simulink model "tenzoRobustV1"  (Simulink 7.9)
settings: Solver=ode23s  StartTime=0.0  StopTime=15  RelTol=1e-3
values from neighbouring files (symbols this model uses):
  AMI = AK1    [AstaTenzoV3.m]
  AMin = [ ... (first row only)    [AstaTenzoV3.m]
  Aoss = AMin-V*ClocalMin    [AstaTenzoV3.m]
  BMI = BK1    [AstaTenzoV3.m]
  ClocalMin = [ ... (first row only)    [AstaTenzoV3.m]
  CMI = eye(q*mu)    [AstaTenzoV3.m]
  Coss = eye(n)    [AstaTenzoV3.m]
  D_phi = [1 325.437715018286 23852.1596168943 0]    [AstaTenzoV3.m]
  D_psi = [1 378.139322580724 35127.9961825618 0]    [AstaTenzoV3.m]
  D_theta = [1 325.437715018286 23852.1596168943 0]    [AstaTenzoV3.m]
  D_thrust = [1 963.786798861645 190423.384445206 0]    [AstaTenzoV3.m]
  DMI = zeros(q*mu,q)    [AstaTenzoV3.m]
  Dmod = [N D]    [AstaTenzoV3.m]
  Doss = zeros(size(Bossw))    [AstaTenzoV3.m]
  F1 = F(:,size(AMin,1)+1:size(F,2))    [AstaTenzoV3.m]
  F2 = F(:,1:size(AMin,1))    [AstaTenzoV3.m]
  k1 = 1    [AstaTenzoV3.m]
  k2 = 1.869    [AstaTenzoV3.m]
  k3 = 2.002    [AstaTenzoV3.m]
  k4 = 1.996    [AstaTenzoV3.m]
  Kt = ct*rho*rp^4*pi()    [AstaTenzoV3.m]
  Ktm = Km/Kt    [AstaTenzoV3.m]
  lx = 28.8e-3    (= 0.0288)    [AstaTenzoV3.m]
  ly = 28.8e-3    (= 0.0288)    [AstaTenzoV3.m]
  N_phi = [440.513056398418 26779.6272064186          272303.182447317 584729.91630594]    [AstaTenzoV3.m]
  N_psi = [59260.0621820611 3429565.45270113           27702908.9364068 53625940.9126871]    [AstaTenzoV3.m]
  N_theta = [440.513056398418 26779.6272064186          272303.182447317 584729.91630594]    [AstaTenzoV3.m]
  N_thrust = [682900.887332905 4668183.15145263]    [AstaTenzoV3.m]
  omega = 0.5    [AstaTenzoV3.m]
  tc = 0.436    [AstaTenzoV3.m]
undefined symbols (not defined in the file or in its folder): Bmod, Boss, EasyHardSat, magnitude, satMaxRPM, satMenoW, satNegThrust, satTau, satThrust, satW
libraries: simulink x4
settings Model: Creator=danilo  LastModifiedBy=userk
settings DebuggingCC: FcnCallInpInsideContextMsg=Use local settings
settings GRTTargetCC: CombineOutputUpdateFcns=off  GRTInterface=on

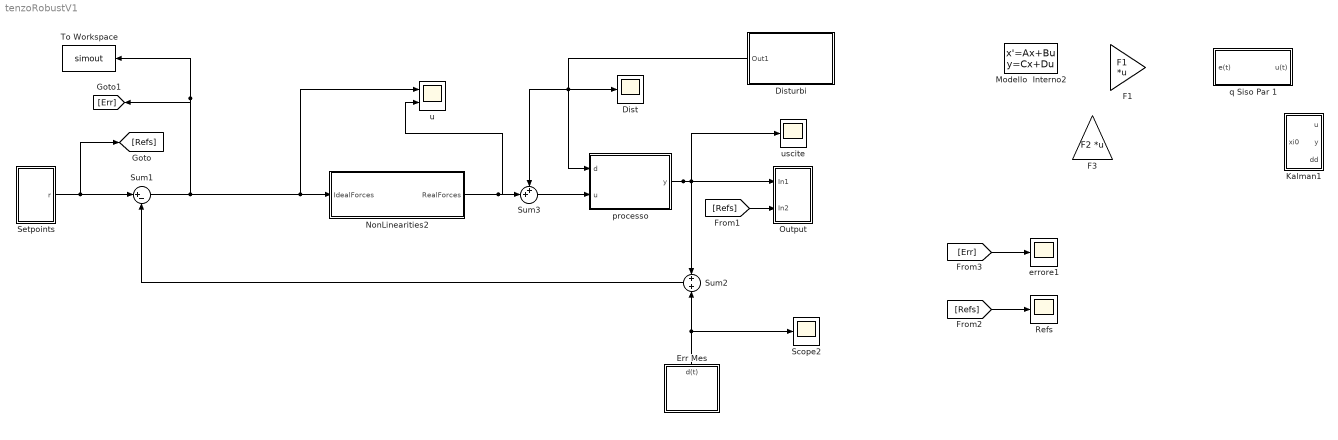
== system tenzoRobustV1 ==
  Dist : Scope
      settings: TimeRange=15  YMin=-0.1  YMax=0.09  SaveName=ScopeData22
  Disturbi : Subsystem
  Err Mes : Subsystem
  F1 : Gain  Gain=F1  Multiplication=Matrix(K*u) (u vector)
  F3 : Gain  Gain=F2  Multiplication=Matrix(K*u) (u vector)
  Kalman1 : Subsystem
  Modello  Interno2 : StateSpace  A=AMI  B=BMI  C=CMI  D=DMI
  NonLinearities2 : Subsystem
  Output : Subsystem
  Refs : Scope
  Scope2 : Scope
      settings: YMin=-0.004  YMax=0.004  SaveName=ScopeData21
  Setpoints : Subsystem
  Sum1 : Sum  Inputs=|+-
  Sum2 : Sum  Inputs=+|+
  Sum3 : Sum  Inputs=++|
  To Workspace : ToWorkspace  VariableName=simout  SampleTime=-1  SaveFormat=Structure
  errore1 : Scope
      settings: SaveName=ScopeData8
  processo : Subsystem
  q Siso Par 1 : Subsystem
  u : Scope  NumInputPorts=2
      settings: YMin=-5~-5  YMax=5~5  SaveName=ScopeData3
  uscite : Scope
      settings: TimeRange=15  YMin=1.3  YMax=2.6  SaveName=ScopeData2
  wires:
  Setpoints/1(r) -> Sum1/1, [Refs]
  processo/1(y) -> Output/1(In1), uscite/1, Sum2/1
  Sum1/1 -> To Workspace/1, [Err], u/1, NonLinearities2/1(IdealForces)
  [Refs] -> Output/2(In2)
  [Refs] -> Refs/1
  [Err] -> errore1/1
  Err Mes/1("  d(t)") -> Sum2/2, Scope2/1
  Sum2/1 -> Sum1/2
  Disturbi/1(Out1) -> processo/1(d), Dist/1, Sum3/1
  Sum3/1 -> processo/2(u)
  NonLinearities2/1(RealForces) -> Sum3/2, u/2

== system tenzoRobustV1/Disturbi ==
  Disturbi Hard : Subsystem
  DisturboEasy : Subsystem
  Manual Switch : simulink/Signal Routing/Manual Switch  sw=1  action=0  varsize=off
  Out1 : Outport
  wires:
  DisturboEasy/1(Out1) -> Manual Switch/1
  Disturbi Hard/1("  d(t)") -> Manual Switch/2
  Manual Switch/1 -> Out1/1

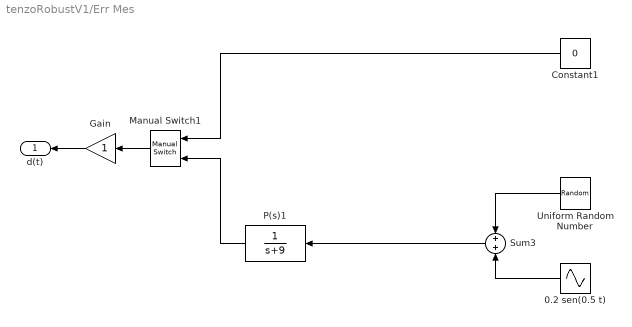
== system tenzoRobustV1/Err Mes ==
  0.2 sen(0.5 t) : Sin  Amplitude=0.02  Frequency=50  Phase=1  SampleTime=0
  Constant1 : Constant  Value=0
  Gain : Gain
  Manual Switch1 : simulink/Signal Routing/Manual Switch  sw=1  action=0  varsize=off
  P(s)1 : TransferFcn  Numerator=1  Denominator=[1 9]
  Sum3 : Sum
  Uniform Random Number : UniformRandomNumber  Minimum=-0.05  Maximum=0.05  SampleTime=0.1
  "  d(t)" : Outport
  wires:
  Uniform Random Number/1 -> Sum3/1
  0.2 sen(0.5 t)/1 -> Sum3/2
  Sum3/1 -> P(s)1/1
  Constant1/1 -> Manual Switch1/1
  P(s)1/1 -> Manual Switch1/2
  Gain/1 -> "  d(t)"/1
  Manual Switch1/1 -> Gain/1

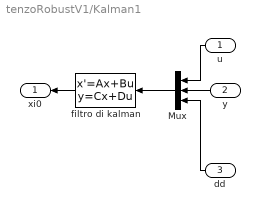
== system tenzoRobustV1/Kalman1 ==
  u : Inport
  y : Inport  Port=2
  dd : Inport  Port=3
  Mux : Mux  Inputs=[4 4 1]
  filtro di kalman : StateSpace  A=Aoss  B=Boss  C=Coss  D=Doss
  xi0 : Outport
  wires:
  dd/1 -> Mux/3
  y/1 -> Mux/2
  filtro di kalman/1 -> xi0/1
  u/1 -> Mux/1
  Mux/1 -> filtro di kalman/1

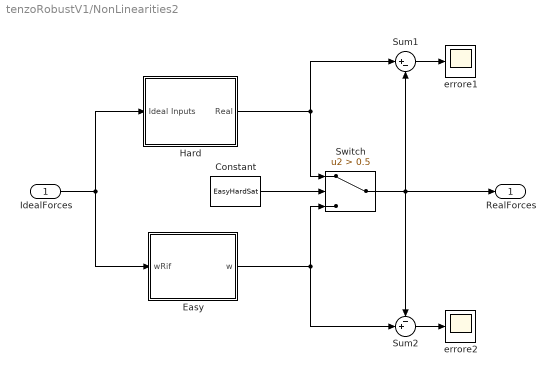
== system tenzoRobustV1/NonLinearities2 ==
  IdealForces : Inport
  Constant : Constant  Value=EasyHardSat
  Easy : Subsystem
  Hard : Subsystem
  Sum1 : Sum  Inputs=|+-
  Sum2 : Sum  Inputs=-+|
  Switch : Switch  Criteria=u2 > Threshold  Threshold=0.5
  errore1 : Scope
      settings: SaveName=ScopeData18
  errore2 : Scope
      settings: SaveName=ScopeData20
  RealForces : Outport
  wires:
  Sum2/1 -> errore2/1
  Sum1/1 -> errore1/1
  IdealForces/1 -> Easy/1(wRif), Hard/1(Ideal Inputs)
  Hard/1(Real) -> Sum1/1, Switch/1
  Easy/1(w) -> Sum2/2, Switch/3
  Switch/1 -> Sum2/1, Sum1/2, RealForces/1
  Constant/1 -> Switch/2

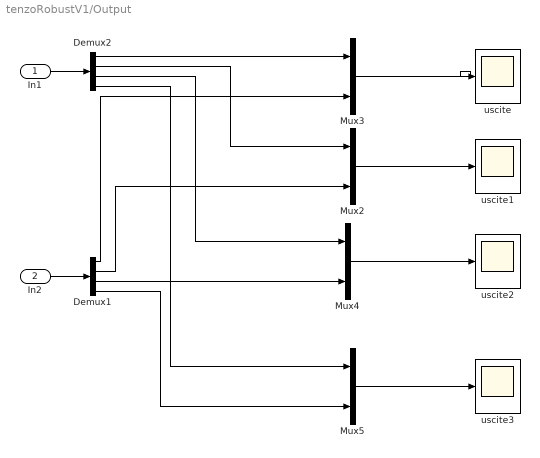
== system tenzoRobustV1/Output ==
  In1 : Inport
  In2 : Inport  Port=2
  Demux1 : Demux
  Demux2 : Demux
  Mux{2..5} (4 alike) : Mux  Inputs=2
  uscite{,1..3} (4 alike) : Scope
      uscite settings: TickLabels=on  TimeRange=15  YMin=-3.5  YMax=7
      uscite1 settings: TickLabels=on  TimeRange=30  YMin=0.75  YMax=4.25  SaveName=ScopeData4
      uscite2 settings: TickLabels=on  YMin=0.75  YMax=4.25  SaveName=ScopeData6
      uscite3 settings: TickLabels=on  YMin=0.75  YMax=4.25  SaveName=ScopeData7
  wires:
  Demux1/1 -> Mux3/2
  In2/1 -> Demux1/1
  In1/1 -> Demux2/1
  Mux3/1 -> uscite/1
  Demux2/1 -> Mux3/1
  Mux2/1 -> uscite1/1
  Demux2/2 -> Mux2/1
  Mux4/1 -> uscite2/1
  Demux2/3 -> Mux4/1
  Mux5/1 -> uscite3/1
  Demux2/4 -> Mux5/1
  Demux1/2 -> Mux2/2
  Demux1/3 -> Mux4/2
  Demux1/4 -> Mux5/2

== system tenzoRobustV1/Setpoints ==
  Mux : Mux  Inputs=[1 1 1 1]
  PsiRef : Step  Time=0.8  After=2.5  SampleTime=0
  ThetRef : Step  Time=0.5  After=2  SampleTime=0
  ZRef : Step  Time=3  After=2.5  SampleTime=0
  phiRef : Step  After=1.5  SampleTime=0
  r : Outport
  wires:
  Mux/1 -> r/1
  phiRef/1 -> Mux/1
  ThetRef/1 -> Mux/2
  PsiRef/1 -> Mux/3
  ZRef/1 -> Mux/4

== system tenzoRobustV1/processo ==
  d : Inport
  u : Inport  Port=2
  Mux : Mux  Inputs=[1 4]
  Processo1 : StateSpace  A=AMin  B=Bmod  C=ClocalMin  D=Dmod
  y : Outport
  wires:
  Mux/1 -> Processo1/1
  d/1 -> Mux/1
  Processo1/1 -> y/1
  u/1 -> Mux/2

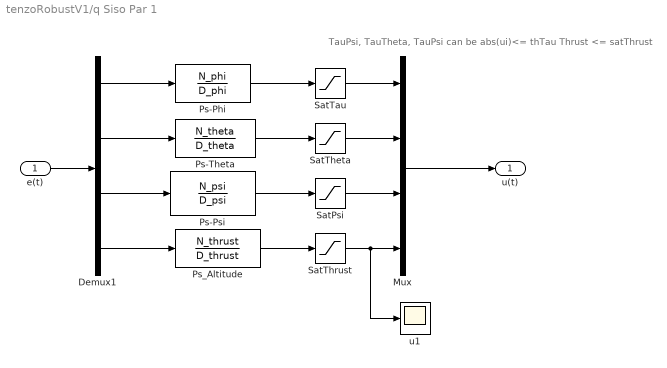
== system tenzoRobustV1/q Siso Par 1 ==
  note: TauPsi, TauTheta, TauPsi
      |  can be abs(ui)<= thTau
      | Thrust <= satThrust
  e(t) : Inport
  Demux1 : Demux
  Mux : Mux
  Ps-Phi : TransferFcn  Numerator=N_phi  Denominator=D_phi
  Ps-Psi : TransferFcn  Numerator=N_psi  Denominator=D_psi
  Ps-Theta : TransferFcn  Numerator=N_theta  Denominator=D_theta
  Ps_Altitude : TransferFcn  Numerator=N_thrust  Denominator=D_thrust
  SatPsi : Saturate  UpperLimit=satTau  LowerLimit=-satTau
  SatTau : Saturate  UpperLimit=satTau  LowerLimit=-satTau
  SatTheta : Saturate  UpperLimit=satTau  LowerLimit=-satTau
  SatThrust : Saturate  UpperLimit=satThrust  LowerLimit=-satNegThrust
  u1 : Scope
      settings: SaveName=ScopeData9
  u(t) : Outport
  wires:
  SatTau/1 -> Mux/1
  SatTheta/1 -> Mux/2
  SatPsi/1 -> Mux/3
  SatThrust/1 -> u1/1, Mux/4
  Demux1/1 -> Ps-Phi/1
  Demux1/3 -> Ps-Psi/1
  Demux1/4 -> Ps_Altitude/1
  Ps-Phi/1 -> SatTau/1
  Ps_Altitude/1 -> SatThrust/1
  Demux1/2 -> Ps-Theta/1
  Ps-Theta/1 -> SatTheta/1
  Ps-Psi/1 -> SatPsi/1
  e(t)/1 -> Demux1/1
  Mux/1 -> u(t)/1

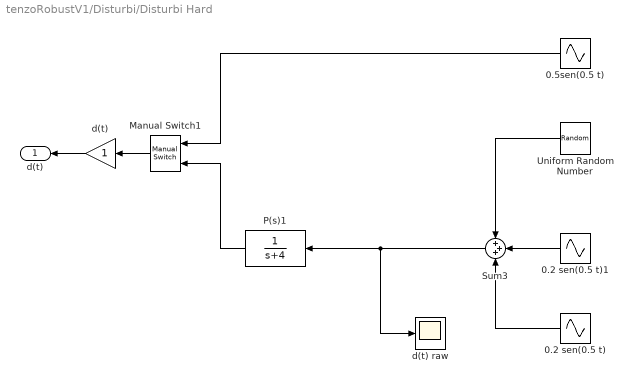
== system tenzoRobustV1/Disturbi/Disturbi Hard ==
  0.2 sen(0.5 t) : Sin  Amplitude=0.2  Frequency=0.5  Phase=1  SampleTime=0
  0.2 sen(0.5 t)1 : Sin  Amplitude=0.1  Frequency=1.5  Phase=1.5  SampleTime=0
  0.5sen(0.5 t) : Sin  Amplitude=0.5  Frequency=0.5  Phase=1  SampleTime=0
  Manual Switch1 : simulink/Signal Routing/Manual Switch  sw=0  action=0  varsize=off
  P(s)1 : TransferFcn  Numerator=1  Denominator=[1 4]
  Sum3 : Sum  Inputs=+++
  Uniform Random Number : UniformRandomNumber  Minimum=-0.5  Maximum=0.5  SampleTime=0.1
  d(t) : Gain
  d(t) raw : Scope
      settings: TimeRange=15  YMin=-0.65  YMax=0.05  SaveName=ScopeData24
  "  d(t)" : Outport
  wires:
  Uniform Random Number/1 -> Sum3/1
  0.2 sen(0.5 t)/1 -> Sum3/3
  Sum3/1 -> P(s)1/1, d(t) raw/1
  0.5sen(0.5 t)/1 -> Manual Switch1/1
  P(s)1/1 -> Manual Switch1/2
  d(t)/1 -> "  d(t)"/1
  Manual Switch1/1 -> d(t)/1
  0.2 sen(0.5 t)1/1 -> Sum3/2

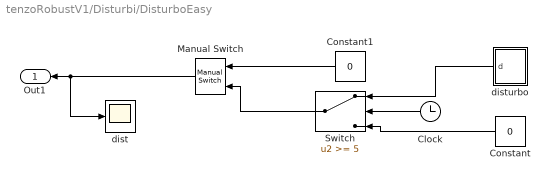
== system tenzoRobustV1/Disturbi/DisturboEasy ==
  Clock : Clock
  Constant : Constant  Value=0
  Constant1 : Constant  Value=0
  Manual Switch : simulink/Signal Routing/Manual Switch  sw=1  action=0  varsize=off
  Switch : Switch  Threshold=5
  dist : Scope
      settings: SaveName=ScopeData5
  disturbo : Subsystem
  Out1 : Outport
  wires:
  Clock/1 -> Switch/2
  disturbo/1(d) -> Switch/1
  Constant/1 -> Switch/3
  Constant1/1 -> Manual Switch/1
  Switch/1 -> Manual Switch/2
  Manual Switch/1 -> dist/1, Out1/1

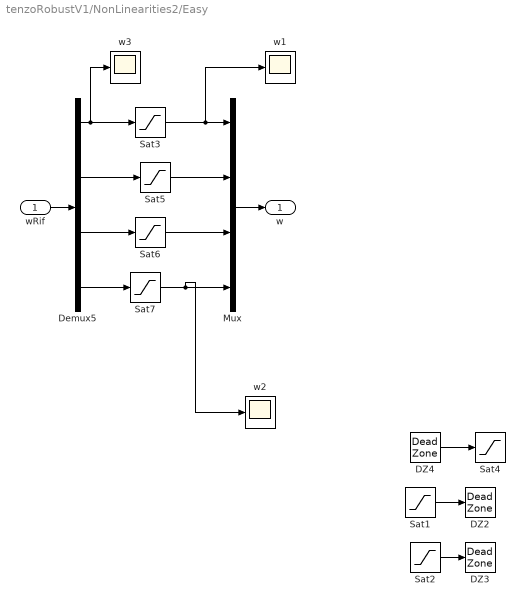
== system tenzoRobustV1/NonLinearities2/Easy ==
  wRif : Inport
  DZ2 : DeadZone  LowerValue=0  UpperValue=deadMotorsZone  SaturateOnIntegerOverflow=on
  DZ3 : DeadZone  LowerValue=0  UpperValue=deadMotorsZone  SaturateOnIntegerOverflow=on
  DZ4 : DeadZone  LowerValue=0  UpperValue=deadMotorsZone  SaturateOnIntegerOverflow=on
  Demux5 : Demux
  Mux : Mux
  Sat1 : Saturate  UpperLimit=satMaxRPM  LowerLimit=0
  Sat2 : Saturate  UpperLimit=satMaxRPM  LowerLimit=0
  Sat{3,5..7} (4 alike) : Saturate  UpperLimit=satW  LowerLimit=satMenoW
  Sat4 : Saturate  UpperLimit=satMaxRPM  LowerLimit=0
  w1 : Scope
      settings: YMin=-1.5e+42  YMax=2.25e+42  SaveName=ScopeData15
  w2 : Scope
      settings: YMin=-8e+50  YMax=5e+50  SaveName=ScopeData10
  w3 : Scope
      settings: YMin=904.495  YMax=999.705  SaveName=ScopeData16
  w : Outport
  wires:
  Sat2/1 -> DZ3/1
  Sat1/1 -> DZ2/1
  DZ4/1 -> Sat4/1
  Mux/1 -> w/1
  wRif/1 -> Demux5/1
  Demux5/1 -> w3/1, Sat3/1
  Sat3/1 -> w1/1, Mux/1
  Sat5/1 -> Mux/2
  Sat7/1 -> Mux/4, w2/1
  Sat6/1 -> Mux/3
  Demux5/2 -> Sat5/1
  Demux5/3 -> Sat6/1
  Demux5/4 -> Sat7/1

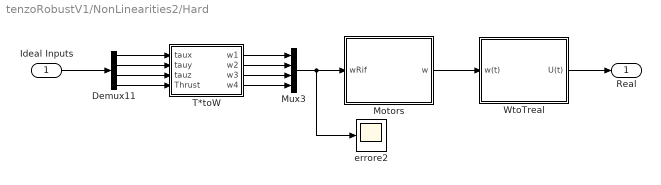
== system tenzoRobustV1/NonLinearities2/Hard ==
  Ideal Inputs : Inport
  Demux11 : Demux
  Motors : Subsystem
  Mux3 : Mux
  T*toW : MATLAB Function  TreatAsAtomicUnit=on
  WtoTreal : Subsystem
  errore2 : Scope
      settings: SaveName=ScopeData23
  Real : Outport
  wires:
  T*toW/4(w4) -> Mux3/4
  T*toW/3(w3) -> Mux3/3
  T*toW/2(w2) -> Mux3/2
  T*toW/1(w1) -> Mux3/1
  Demux11/4 -> T*toW/4(Thrust)
  Demux11/3 -> T*toW/3(tauz)
  Demux11/2 -> T*toW/2(tauy)
  Demux11/1 -> T*toW/1(taux)
  Motors/1(w) -> WtoTreal/1(w(t))
  Mux3/1 -> Motors/1(wRif), errore2/1
  Ideal Inputs/1 -> Demux11/1
  WtoTreal/1(U(t)) -> Real/1

== system tenzoRobustV1/Disturbi/DisturboEasy/disturbo ==
  Constant : Constant
  Sine Wave : Sin  Amplitude=0.5  Frequency=omega  SampleTime=0
  Sum2 : Sum  Inputs=|++
  d : Outport
  wires:
  Sine Wave/1 -> Sum2/2
  Constant/1 -> Sum2/1
  Sum2/1 -> d/1

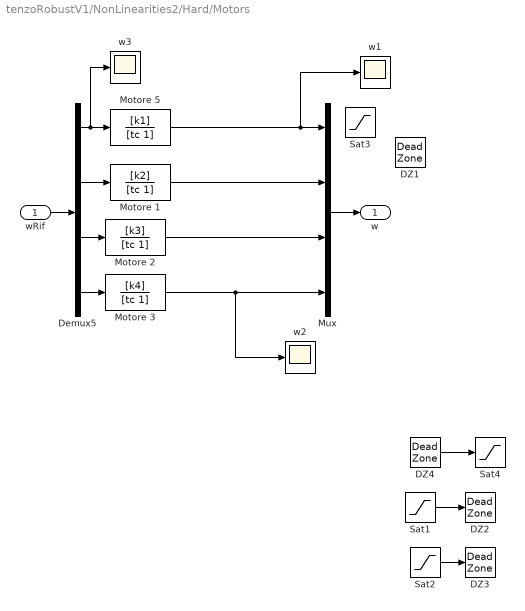
== system tenzoRobustV1/NonLinearities2/Hard/Motors ==
  wRif : Inport
  DZ{1..4} (4 alike) : DeadZone  LowerValue=0  UpperValue=deadMotorsZone  SaturateOnIntegerOverflow=on
  Demux5 : Demux
  Motore 1 : TransferFcn  Numerator=[k2]  Denominator=[tc 1]
  Motore 2 : TransferFcn  Numerator=[k3]  Denominator=[tc 1]
  Motore 3 : TransferFcn  Numerator=[k4]  Denominator=[tc 1]
  Motore 5 : TransferFcn  Numerator=[k1]  Denominator=[tc 1]
  Mux : Mux
  Sat{1..4} (4 alike) : Saturate  UpperLimit=satMaxRPM  LowerLimit=0
  w1 : Scope
      settings: YMin=-1.5e+42  YMax=2.25e+42  SaveName=ScopeData15
  w2 : Scope
      settings: YMin=-8e+50  YMax=5e+50  SaveName=ScopeData10
  w3 : Scope
      settings: YMin=904.495  YMax=999.705  SaveName=ScopeData16
  w : Outport
  wires:
  Demux5/1 -> Motore 5/1, w3/1
  Demux5/2 -> Motore 1/1
  Demux5/3 -> Motore 2/1
  Demux5/4 -> Motore 3/1
  wRif/1 -> Demux5/1
  Mux/1 -> w/1
  Motore 5/1 -> Mux/1, w1/1
  Motore 1/1 -> Mux/2
  Motore 2/1 -> Mux/3
  Motore 3/1 -> Mux/4, w2/1
  DZ4/1 -> Sat4/1
  Sat1/1 -> DZ2/1
  Sat2/1 -> DZ3/1

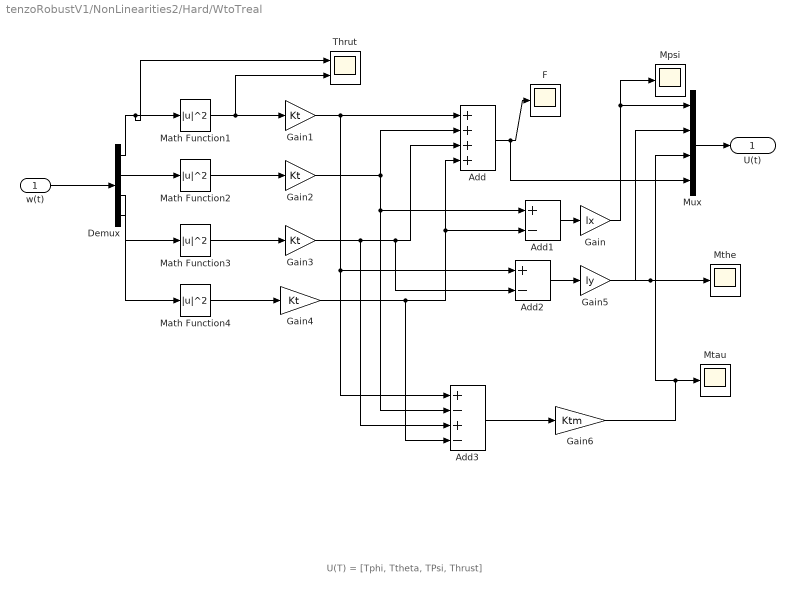
== system tenzoRobustV1/NonLinearities2/Hard/WtoTreal ==
  note: U(T) = [Tphi, Ttheta, TPsi, Thrust]
  w(t) : Inport
  Add : Sum  Inputs=++++
  Add1 : Sum  Inputs=+-
  Add2 : Sum  Inputs=+-
  Add3 : Sum  Inputs=+-+-
  Demux : Demux
  F : Scope
      settings: SaveName=ScopeData17
  Gain : Gain  Gain=lx
  Gain{1..4} (4 alike) : Gain  Gain=Kt
  Gain5 : Gain  Gain=ly
  Gain6 : Gain  Gain=Ktm
  Math Function{1..4} (4 alike) : Math  Operator=magnitude^2  SaturateOnIntegerOverflow=on
  Mpsi : Scope
      settings: SaveName=ScopeData14
  Mtau : Scope
      settings: SaveName=ScopeData11
  Mthe : Scope
      settings: SaveName=ScopeData13
  Mux : Mux
  Thrut : Scope  NumInputPorts=2
      settings: YMin=-5~-5  YMax=5~5  SaveName=ScopeData19
  U(t) : Outport
  wires:
  w(t)/1 -> Demux/1
  Demux/4 -> Math Function4/1
  Demux/3 -> Math Function3/1
  Mux/1 -> U(t)/1
  Demux/2 -> Math Function2/1
  Demux/1 -> Thrut/1, Math Function1/1
  Gain6/1 -> Mtau/1, Mux/3
  Add3/1 -> Gain6/1
  Gain5/1 -> Mthe/1, Mux/2
  Gain/1 -> Mpsi/1, Mux/1
  Add2/1 -> Gain5/1
  Add1/1 -> Gain/1
  Add/1 -> F/1, Mux/4
  Gain4/1 -> Add3/4, Add1/2, Add/4
  Gain3/1 -> Add3/3, Add2/2, Add/3
  Gain2/1 -> Add3/2, Add1/1, Add/2
  Gain1/1 -> Add3/1, Add2/1, Add/1
  Math Function4/1 -> Gain4/1
  Math Function3/1 -> Gain3/1
  Math Function2/1 -> Gain2/1
  Math Function1/1 -> Thrut/2, Gain1/1

== matlab function NonLinearities2/Hard/T*toW ==
  data: taux input double; tauy input double; tauz input double; Thrust input double; w1 output double; w2 output double; w3 output double; w4 output double
function [w1,w2,w3,w4] = mixer(taux,tauy,tauz,Thrust)
%#codegen
%% Physical properties of the environment
g=9.81; %Acceleration of gravity (m)
rho=1.2; %Density of air (m^3.kg^-1)

%% Physical properties of the quadrotor

% Total mass of the quadrotor [Kg]
mq=0.82;
% Motor length along x-axis (m). All motors have equal sizes.
lx=28.8e-3;
% Motor length along y-axis (m)
ly=28.8e-3;
% Motor length along z-axis (m)
lz=26e-3;

% Distance from the center of gravity to the center of a motor (m).
% The quadrotor is symmetric regarding the XZ and YZ planes, so
% dcg is the same for all motors.
dcg=0.288; 


% Inflow coefficient
If = -0.3559;

% Thrust coefficient of the propeller and Power coefficient
cp=0.0743; 
ct=0.1154;

% Propeller radius (m)
rp=25.4e-3; 
% Constant value to calculate the moment provided
% by a propeller given its angular speed (kg.m^2.rad^-1)
Km=cp*4*rho*rp^5/pi()^3; 
% Constant value to calculate the thrust provided
% by a propeller given its angular speed (kg.m.rad^-1) 
%Kt=ct*4*rho*rp^4/pi()^2; 
Kt=ct*rho*rp^2*pi();
% Constant that relates thrust and moment of a propeller.
Ktm=Km/Kt;
k1=2.028; %Transfer-function gain of motor 1
k2=1.869; %Transfer-function gain of motor 2
k3=2.002; %Transfer-function gain of motor 3
k4=1.996; %Transfer-function gain of motor 4
tc=0.436; %Time-constant of the motors (assumed equal for all motors)

dz1=1247.4; %PWM dead-zone of motor 1 given its first-order transfer
% function (micro-seconds)
dz2=1247.8; % PWM dead-zone of motor 2 given its first-order transfer
%function (micro-seconds)
dz3=1246.4; % PWM dead-zone of motor 3 given its first-order transfer
%function (micro-seconds)
dz4=1247.9; % PWM dead-zone of motor 4 given its first-order transfer
% 
% g_m1=tf(k1,[tc 1]); % First-order transfer-function of motor 1
% g_m2=tf(k2,[tc 1]); % First-order transfer-function of motor 2
% g_m3=tf(k3,[tc 1]); % First-order transfer-function of motor 3
% g_m4=tf(k4,[tc 1]); % First-order transfer-function of motor 4

%vNote: If the behavior of the motors is not linear, linearization around
% an operating point is required to attain these transfer-functions.
PWM_max=2200; %Upper limit of the PWM signal provided to
%the motors (micro-seconds)
w0c=sqrt(g*mq/Kt);
%X0c=w0c;
Ft0=mq*g;


%% u=[T; taux; tauy; tauz];

% WTF = [ -Kt -Kt -Kt -Kt;
%          0   -lx*Kt  0  lx*Kt;
%         ly*Kt  0  -ly*Kt  0;
%         Ktm -Ktm Ktm -Ktm];   
%    T= WTF^(-1)*[Thrust; taux; tauy; tauz];

%%  u=[taux; tauy; tauz, T];

WTF = [     0   -lx*Kt  0  lx*Kt;
            ly*Kt  0  -ly*Kt  0;
            Ktm -Ktm Ktm -Ktm;
            -Kt -Kt -Kt -Kt];   

WTFm1 = WTF^(-1);
T= WTFm1*[taux; tauy; tauz; Thrust];

%% Conversion

    w1 = T(1);
    w2 = T(2);
    w3 = T(3);
    w4 = T(4);
